simulink model "Test_of_Hover_Controller"  (R2023a)
settings: Solver=FixedStepAuto  StartTime=0.0  StopTime=150  FixedStep=0.001  RelTol=1e-3
libraries: simulink x2
settings Model: Creator=邓宇飞  LastModifiedBy=邓宇飞

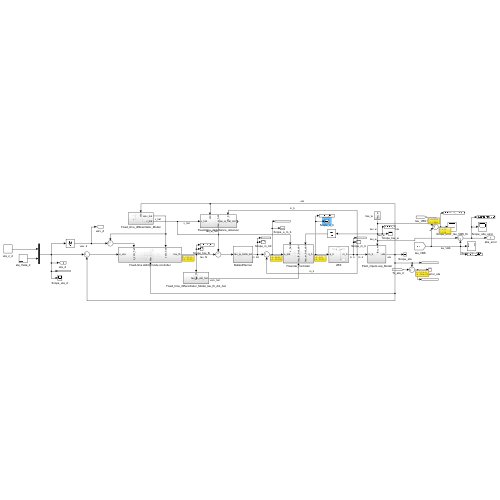
[thumbnail: Simulink's stored preview of the top-level diagram]
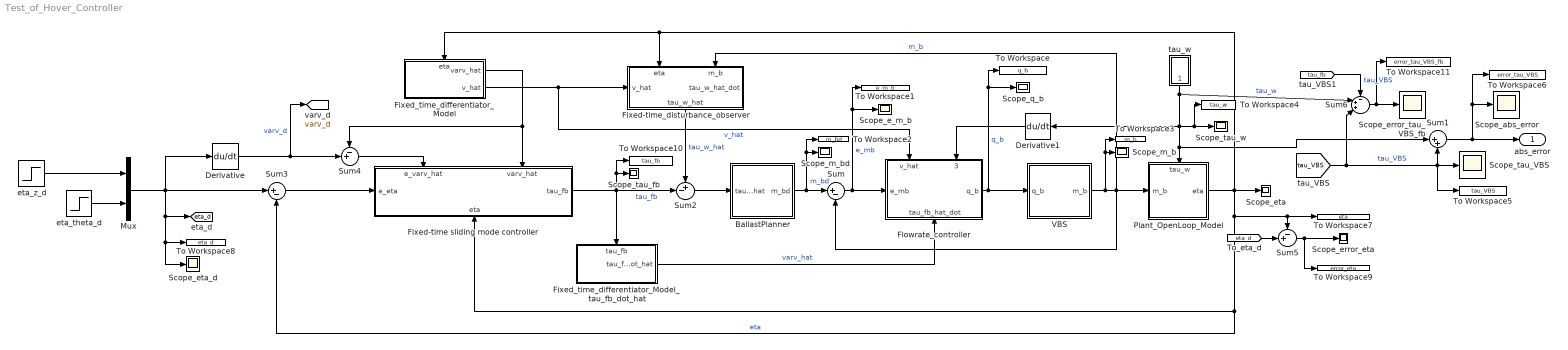
== system Test_of_Hover_Controller ==
  BallastPlanner : Subsystem
  Derivative : Derivative
  Derivative1 : Derivative
  Fixed-time sliding mode controller : Subsystem
      settings: PortSchema="{\"entries\":[{\"content\":{\"sides\":[{\"content\":{\"connectorIds\":[\"In1\"]},\"type\":\"ConnectorPlacement.EquallySpacedRectSide\",\"uuid\":\"f7eec32a-11e5-493e-91a4-aa23e7798835\"},{\"content\":{\"connectorIds\":[\"Out1\"],\"side\":\"RIGHT\"},\"type\":\"ConnectorPlacement.EquallySpacedRectSide\",\"uuid\":\"2b78eec5-73c8-4d02-9319-0fb2d1bcee33\"},{\"content\":{\"connectorIds\":[\"In2\",\"In3\"],\"side\":\"TOP\"},\"type\":\"ConnectorPlacement.EquallySpacedRectSide\",\"uuid\":\"6bb67a89-6549-4a25-872d-286d7aa8440b\"},{\"content\":{\"connectorIds\":[\"In4\"],\"side\":\"BOTTOM\"},\"type\":\"ConnectorPlacement.EquallySpacedRectSide\",\"uuid\":\"a7c480fa-a393-4283-926e-8262b2c36ba1\"}]},\"type\":\"ConnectorPlacement.EquallySpacedConnector\",\"uuid\":\"ac88fafb-ad61-4f2d-a744-8be38b32af3c\"}],\"packageUris\":[\"http://schema.mathworks.com/mf0/Connector/R2020b\"],\"version\":\"1.0\"}"
  Fixed-time_disturbance_observer : Subsystem
      settings: PortSchema="{\"entries\":[{\"content\":{\"sides\":[{\"content\":{\"connectorIds\":[\"In1\"]},\"type\":\"ConnectorPlacement.EquallySpacedRectSide\",\"uuid\":\"977a3149-1921-48fe-b96a-a4ad28c91371\"},{\"content\":{\"connectorIds\":[\"Out1\"],\"side\":\"RIGHT\"},\"type\":\"ConnectorPlacement.EquallySpacedRectSide\",\"uuid\":\"fff94096-65c1-4681-8bdf-eed371b61c52\"},{\"content\":{\"connectorIds\":[\"In2\",\"In3\"],\"side\":\"TOP\"},\"type\":\"ConnectorPlacement.EquallySpacedRectSide\",\"uuid\":\"5bed714d-ab4b-433b-a946-feaea2816cb1\"},{\"content\":{\"connectorIds\":[\"Out2\"],\"side\":\"BOTTOM\"},\"type\":\"ConnectorPlacement.EquallySpacedRectSide\",\"uuid\":\"4ad85521-d335-4ab1-88b6-9b8c0a3b2785\"}]},\"type\":\"ConnectorPlacement.EquallySpacedConnector\",\"uuid\":\"7c33b186-f768-465e-b799-f94ef9fdf411\"}],\"packageUris\":[\"http://schema.mathworks.com/mf0/Connector/R2020b\"],\"version\":\"1.0\"}"
  Fixed_time_differentiator_Model : Subsystem
      settings: PortSchema="{\"entries\":[{\"content\":{\"sides\":[{\"content\":{},\"type\":\"ConnectorPlacement.EquallySpacedRectSide\",\"uuid\":\"99f788c9-d3b5-4afa-bbaa-ac2c57ad12cb\"},{\"content\":{\"connectorIds\":[\"Out1\",\"Out2\"],\"side\":\"RIGHT\"},\"type\":\"ConnectorPlacement.EquallySpacedRectSide\",\"uuid\":\"b4add6d1-b599-4d1a-a211-146e19e09e31\"},{\"content\":{\"connectorIds\":[\"In1\"],\"side\":\"TOP\"},\"type\":\"ConnectorPlacement.EquallySpacedRectSide\",\"uuid\":\"d4aeca70-b9bd-44c3-bfe7-6ab0567a3ae9\"}]},\"type\":\"ConnectorPlacement.EquallySpacedConnector\",\"uuid\":\"acaab675-7958-4b63-89da-846c50cb8508\"}],\"packageUris\":[\"http://schema.mathworks.com/mf0/Connector/R2020b\"],\"version\":\"1.0\"}"
  Fixed_time_differentiator_Model_tau_fb_dot_hat : Subsystem
      settings: PortSchema="{\"entries\":[{\"content\":{\"sides\":[{\"content\":{},\"type\":\"ConnectorPlacement.EquallySpacedRectSide\",\"uuid\":\"509b689f-cae1-4523-9372-2499bd3b7d9d\"},{\"content\":{\"connectorIds\":[\"Out1\"],\"side\":\"RIGHT\"},\"type\":\"ConnectorPlacement.EquallySpacedRectSide\",\"uuid\":\"a1df743b-e6a9-4451-86f2-27990c18dc24\"},{\"content\":{\"connectorIds\":[\"In1\"],\"side\":\"TOP\"},\"type\":\"ConnectorPlacement.EquallySpacedRectSide\",\"uuid\":\"5149f091-ad88-4d80-a39f-36dd9d24fd7a\"},{\"content\":{\"side\":\"BOTTOM\"},\"type\":\"ConnectorPlacement.EquallySpacedRectSide\",\"uuid\":\"b5eefe9f-7883-4d8e-a8af-dce689347657\"}]},\"type\":\"ConnectorPlacement.EquallySpacedConnector\",\"uuid\":\"61175d6f-7ec4-4947-9258-193f13282eb9\"}],\"packageUris\":[\"http://schema.mathworks.com/mf0/Connector/R2020b\"],\"version\":\"1.0\"}"
  Flowrate_controller : Subsystem
      settings: PortSchema="{\"entries\":[{\"content\":{\"sides\":[{\"content\":{\"connectorIds\":[\"In1\"]},\"type\":\"ConnectorPlacement.EquallySpacedRectSide\",\"uuid\":\"977a3149-1921-48fe-b96a-a4ad28c91371\"},{\"content\":{\"connectorIds\":[\"Out1\"],\"side\":\"RIGHT\"},\"type\":\"ConnectorPlacement.EquallySpacedRectSide\",\"uuid\":\"fff94096-65c1-4681-8bdf-eed371b61c52\"},{\"content\":{\"connectorIds\":[\"In2\",\"In3\"],\"side\":\"TOP\"},\"type\":\"ConnectorPlacement.EquallySpacedRectSide\",\"uuid\":\"5bed714d-ab4b-433b-a946-feaea2816cb1\"},{\"content\":{\"connectorIds\":[\"In4\"],\"side\":\"BOTTOM\"},\"type\":\"ConnectorPlacement.EquallySpacedRectSide\",\"uuid\":\"e9124608-fe81-4a90-8a38-d0d96a25662d\"}]},\"type\":\"ConnectorPlacement.EquallySpacedConnector\",\"uuid\":\"7c33b186-f768-465e-b799-f94ef9fdf411\"}],\"packageUris\":[\"http://schema.mathworks.com/mf0/Connector/R2020b\"],\"version\":\"1.0\"}"
  Mux : Mux  Inputs=2
  Plant_OpenLoop_Model : Subsystem
      settings: PortSchema="{\"entries\":[{\"content\":{\"sides\":[{\"content\":{\"connectorIds\":[\"In1\"]},\"type\":\"ConnectorPlacement.EquallySpacedRectSide\",\"uuid\":\"171ab365-2c9c-477f-ab94-6e1b535ce398\"},{\"content\":{\"connectorIds\":[\"Out1\"],\"side\":\"RIGHT\"},\"type\":\"ConnectorPlacement.EquallySpacedRectSide\",\"uuid\":\"68d15153-0085-4baf-9515-c294b6b9b8eb\"},{\"content\":{\"connectorIds\":[\"In2\"],\"side\":\"TOP\"},\"type\":\"ConnectorPlacement.EquallySpacedRectSide\",\"uuid\":\"3f887e7e-8b06-4bf2-b39d-d49324deef58\"},{\"content\":{\"side\":\"BOTTOM\"},\"type\":\"ConnectorPlacement.EquallySpacedRectSide\",\"uuid\":\"0c56d0aa-527a-42c0-aa98-8ee52c9400f1\"}]},\"type\":\"ConnectorPlacement.EquallySpacedConnector\",\"uuid\":\"a8f2799e-4d6b-4adf-9803-c3f607cd4a91\"}],\"packageUris\":[\"http://schema.mathworks.com/mf0/Connector/R2020b\"],\"version\":\"1.0\"}"
  Scope_abs_error : Scope
  Scope_e_m_b : Scope
  Scope_error_eta : Scope
  Scope_error_tau_VBS_fb : Scope
  Scope_eta : Scope
  Scope_eta_d : Scope
  Scope_m_b : Scope
  Scope_m_bd : Scope
  Scope_q_b : Scope
  Scope_tau_VBS : Scope
  Scope_tau_fb : Scope
  Scope_tau_w : Scope
  Sum : Sum  Inputs=|+-
  Sum1 : Sum  Inputs=|++
  Sum2 : Sum  Inputs=+-|
  Sum3 : Sum  Inputs=|+-
  Sum4 : Sum  Inputs=-+|
  Sum5 : Sum  Inputs=-+|
  Sum6 : Sum  Inputs=-++|
  To Workspace : ToWorkspace  VariableName=q_b  SaveFormat=Timeseries  SampleTime=-1
  To Workspace1 : ToWorkspace  VariableName=e_m_b  SaveFormat=Timeseries  SampleTime=-1
  To Workspace10 : ToWorkspace  VariableName=tau_fb  SaveFormat=Timeseries  SampleTime=-1
  To Workspace11 : ToWorkspace  VariableName=error_tau_VBS_fb  SaveFormat=Timeseries  SampleTime=-1
  To Workspace2 : ToWorkspace  VariableName=m_bd  SaveFormat=Timeseries  SampleTime=-1
  To Workspace3 : ToWorkspace  VariableName=m_b  SaveFormat=Timeseries  SampleTime=-1
  To Workspace4 : ToWorkspace  VariableName=tau_w  SaveFormat=Timeseries  SampleTime=-1
  To Workspace5 : ToWorkspace  VariableName=tau_VBS  SaveFormat=Timeseries  SampleTime=-1
  To Workspace6 : ToWorkspace  VariableName=error_tau_VBS  SaveFormat=Timeseries  SampleTime=-1
  To Workspace7 : ToWorkspace  VariableName=eta  SaveFormat=Timeseries  SampleTime=-1
  To Workspace8 : ToWorkspace  VariableName=eta_d  SaveFormat=Timeseries  SampleTime=-1
  To Workspace9 : ToWorkspace  VariableName=error_eta  SaveFormat=Timeseries  SampleTime=-1
  VBS : Subsystem
  eta_theta_d : Step  After=0  SampleTime=0
  eta_z_d : Step  After=0  SampleTime=0
  tau_w : Subsystem
  abs_error : Outport
  tag scope: eta_d=global, varv_d=global
  wires:
  Sum3/1 -> Fixed-time sliding mode controller/1(e_eta)
  eta_theta_d/1 -> Mux/2
  [tau_VBS] -> Sum6/3, Scope_tau_VBS/1, Sum1/2, To Workspace5/1  "tau_VBS"
  eta_z_d/1 -> Mux/1
  Sum/1 -> Flowrate_controller/1(e_mb), To Workspace1/1, Scope_e_m_b/1  "e_mb"
  Fixed_time_differentiator_Model/2(v_hat) -> Flowrate_controller/2(v_hat), Fixed-time_disturbance_observer/1(v_hat)  "v_hat"
  Derivative/1 -> [varv_d], Sum4/2  "varv_d"
  tau_w/1(tau_w) -> Sum6/2, To Workspace4/1, Scope_tau_w/1, Plant_OpenLoop_Model/2(tau_w), Sum1/1, Derivative1/1  "tau_w"
  Sum1/1 -> To Workspace6/1, Scope_abs_error/1, abs_error/1
  VBS/1(m_b) -> To Workspace3/1, Scope_m_b/1, Fixed-time_disturbance_observer/3(m_b), Sum/2, Plant_OpenLoop_Model/1(m_b)  "m_b"
  Flowrate_controller/1(q_b) -> Scope_q_b/1, To Workspace/1, VBS/1(q_b)  "q_b"
  Mux/1 -> Sum3/1, [eta_d], To Workspace8/1, Scope_eta_d/1, Derivative/1
  BallastPlanner/1(m_bd) -> To Workspace2/1, Scope_m_bd/1, Sum/1  "m_bd"
  Fixed-time sliding mode controller/1(tau_fb) -> To Workspace10/1, Scope_tau_fb/1, Fixed_time_differentiator_Model_tau_fb_dot_hat/1(tau_fb), Sum2/2  "tau_fb"
  Fixed-time_disturbance_observer/2(tau_w_hat) -> Sum2/1  "tau_w_hat"
  Sum2/1 -> BallastPlanner/1(tau_w_hat)
  Fixed_time_differentiator_Model_tau_fb_dot_hat/1(tau_fb_dot_hat) -> Flowrate_controller/4(tau_fb_hat_dot)  "varv_hat"
  Plant_OpenLoop_Model/1(eta) -> To Workspace7/1, Sum5/1, Fixed-time sliding mode controller/4(eta), Sum3/2, Scope_eta/1, Fixed_time_differentiator_Model/1(eta), Fixed-time_disturbance_observer/2(eta)  "eta"
  Fixed_time_differentiator_Model/1(varv_hat) -> Fixed-time sliding mode controller/3(varv_hat), Sum4/1
  Sum4/1 -> Fixed-time sliding mode controller/2(e_varv_hat)
  Derivative1/1 -> Flowrate_controller/3(tau_w_hat_dot)
  [eta_d] -> Sum5/2
  Sum5/1 -> To Workspace9/1, Scope_error_eta/1
  [tau_fb] -> Sum6/1  "tau_VBS"
  Sum6/1 -> To Workspace11/1, Scope_error_tau_VBS_fb/1

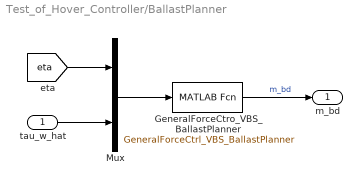
== system Test_of_Hover_Controller/BallastPlanner ==
  tau_w_hat : Inport
  GeneralForceCtro_VBS_BallastPlanner : MATLABFcn  MATLABFcn=GeneralForceCtrl_VBS_BallastPlanner  OutputDimensions=2  OutputSignalType=real
  Mux : Mux  Inputs=2
  m_bd : Outport
  wires:
  Mux/1 -> GeneralForceCtro_VBS_BallastPlanner/1
  GeneralForceCtro_VBS_BallastPlanner/1 -> m_bd/1  "m_bd"
  [eta] -> Mux/1
  tau_w_hat/1 -> Mux/2

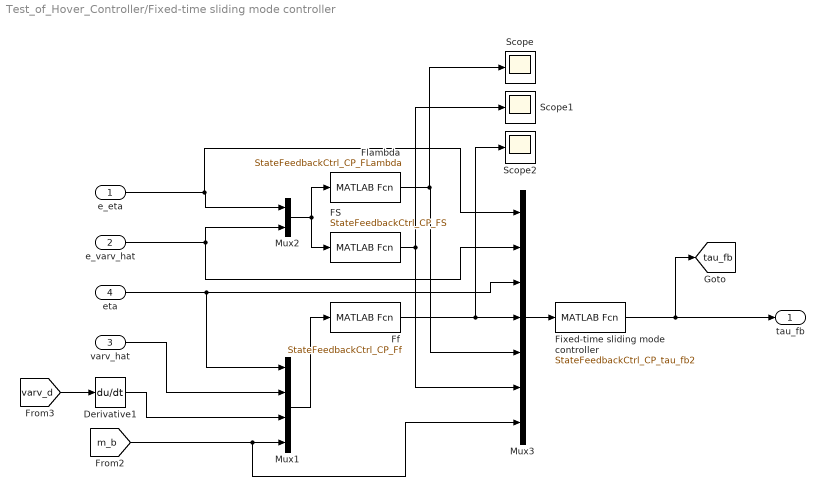
== system Test_of_Hover_Controller/Fixed-time sliding mode controller ==
  e_eta : Inport
  e_varv_hat : Inport  Port=2
  varv_hat : Inport  Port=3
  eta : Inport  Port=4
  Derivative1 : Derivative
  FS : MATLABFcn  MATLABFcn=StateFeedbackCtrl_CP_FS  OutputDimensions=2  OutputSignalType=real
  Ff : MATLABFcn  MATLABFcn=StateFeedbackCtrl_CP_Ff  OutputDimensions=2  OutputSignalType=real
  Fixed-time sliding mode controller : MATLABFcn  MATLABFcn=StateFeedbackCtrl_CP_tau_fb2  OutputDimensions=2  OutputSignalType=real
  Flambda : MATLABFcn  MATLABFcn=StateFeedbackCtrl_CP_FLambda  OutputDimensions=2  OutputSignalType=real
  Mux1 : Mux
  Mux2 : Mux  Inputs=2
  Mux3 : Mux  Inputs=7
  Scope : Scope
  Scope1 : Scope
  Scope2 : Scope
  tau_fb : Outport
  tag scope: tau_fb=global
  wires:
  eta/1 -> Mux3/3, Mux1/1
  e_varv_hat/1 -> Mux2/2, Mux3/2
  e_eta/1 -> Mux3/1, Mux2/1
  Mux2/1 -> Flambda/1, FS/1
  FS/1 -> Scope1/1, Mux3/6
  Flambda/1 -> Scope/1, Mux3/5
  Ff/1 -> Scope2/1, Mux3/4
  Mux1/1 -> Ff/1
  [m_b] -> Mux3/7, Mux1/4
  Mux3/1 -> Fixed-time sliding mode controller/1
  varv_hat/1 -> Mux1/2
  Derivative1/1 -> Mux1/3
  [varv_d] -> Derivative1/1
  Fixed-time sliding mode controller/1 -> tau_fb/1, [tau_fb]

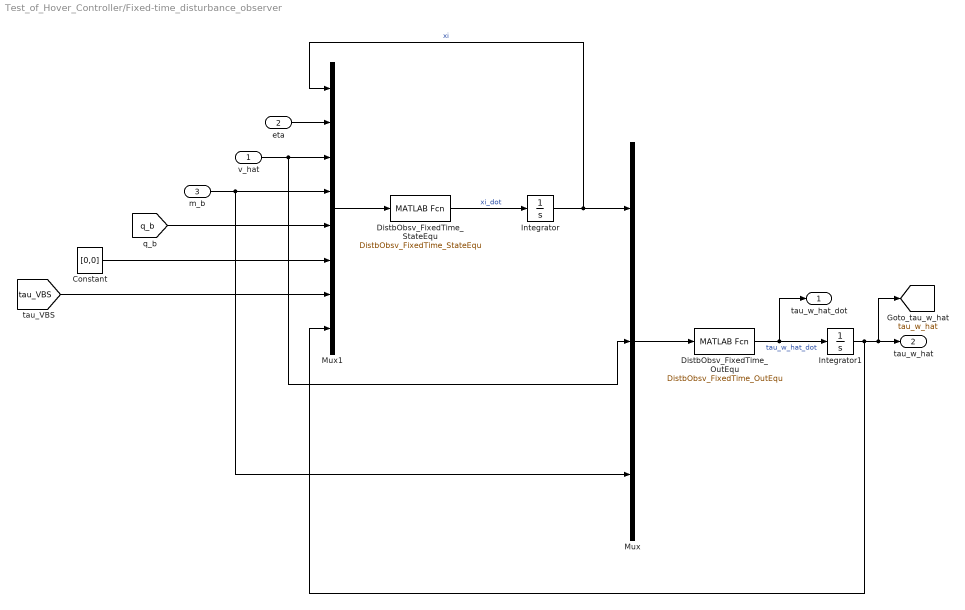
== system Test_of_Hover_Controller/Fixed-time_disturbance_observer ==
  v_hat : Inport
  eta : Inport  Port=2
  m_b : Inport  Port=3
  Constant : Constant  Value=[0,0]
  DistbObsv_FixedTime_OutEqu : MATLABFcn  MATLABFcn=DistbObsv_FixedTime_OutEqu  OutputDimensions=2  OutputSignalType=real
  DistbObsv_FixedTime_StateEqu : MATLABFcn  MATLABFcn=DistbObsv_FixedTime_StateEqu  OutputDimensions=2  OutputSignalType=real
  Integrator : Integrator
  Integrator1 : Integrator
  Mux : Mux  Inputs=3
  Mux1 : Mux  Inputs=8
  tau_w_hat_dot : Outport
  tau_w_hat : Outport  Port=2
  tag scope: tau_w_hat=global
  wires:
  Integrator1/1 -> [tau_w_hat], tau_w_hat/1, Mux1/8
  Integrator/1 -> Mux1/1, Mux/1  "xi"
  DistbObsv_FixedTime_OutEqu/1 -> tau_w_hat_dot/1, Integrator1/1  "tau_w_hat_dot"
  Mux/1 -> DistbObsv_FixedTime_OutEqu/1
  Mux1/1 -> DistbObsv_FixedTime_StateEqu/1
  DistbObsv_FixedTime_StateEqu/1 -> Integrator/1  "xi_dot"
  eta/1 -> Mux1/2
  v_hat/1 -> Mux/2, Mux1/3
  m_b/1 -> Mux/3, Mux1/4
  [q_b] -> Mux1/5
  Constant/1 -> Mux1/6
  [tau_VBS] -> Mux1/7

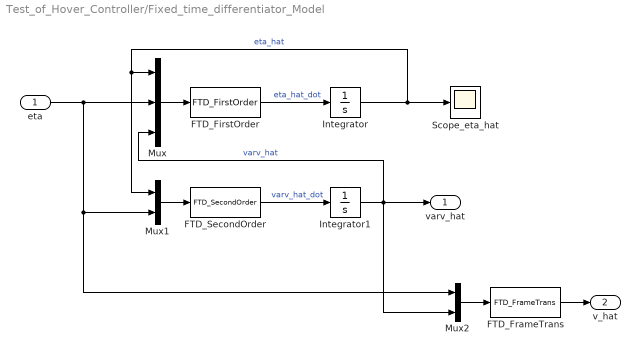
== system Test_of_Hover_Controller/Fixed_time_differentiator_Model ==
  eta : Inport
  FTD_FirstOrder : MATLABFcn  MATLABFcn=FTD_FirstOrder  OutputDimensions=2  OutputSignalType=real
  FTD_FrameTrans : MATLABFcn  MATLABFcn=FTD_FrameTrans  OutputDimensions=2  OutputSignalType=real
  FTD_SecondOrder : MATLABFcn  MATLABFcn=FTD_SecondOrder  OutputDimensions=2  OutputSignalType=real
  Integrator : Integrator
  Integrator1 : Integrator
  Mux : Mux  Inputs=3
  Mux1 : Mux  Inputs=2
  Mux2 : Mux  Inputs=2
  Scope_eta_hat : Scope
  varv_hat : Outport
  v_hat : Outport  Port=2
  wires:
  Integrator1/1 -> Mux2/2, varv_hat/1, Mux/3  "varv_hat"
  eta/1 -> Mux2/1, Mux1/2, Mux/2
  FTD_SecondOrder/1 -> Integrator1/1  "varv_hat_dot"
  FTD_FrameTrans/1 -> v_hat/1
  FTD_FirstOrder/1 -> Integrator/1  "eta_hat_dot"
  Integrator/1 -> Mux1/1, Mux/1, Scope_eta_hat/1  "eta_hat"
  Mux/1 -> FTD_FirstOrder/1
  Mux2/1 -> FTD_FrameTrans/1
  Mux1/1 -> FTD_SecondOrder/1

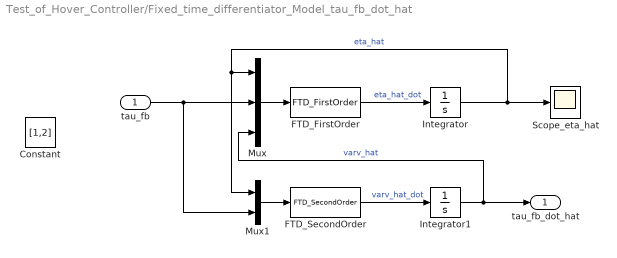
== system Test_of_Hover_Controller/Fixed_time_differentiator_Model_tau_fb_dot_hat ==
  tau_fb : Inport
  Constant : Constant  Value=[1,2]
  FTD_FirstOrder : MATLABFcn  MATLABFcn=FTD_FirstOrder  OutputDimensions=2
  FTD_SecondOrder : MATLABFcn  MATLABFcn=FTD_SecondOrder  OutputDimensions=2
  Integrator : Integrator
  Integrator1 : Integrator
  Mux : Mux  Inputs=3
  Mux1 : Mux  Inputs=2
  Scope_eta_hat : Scope
  tau_fb_dot_hat : Outport
  wires:
  Integrator/1 -> Mux1/1, Mux/1, Scope_eta_hat/1  "eta_hat"
  Integrator1/1 -> tau_fb_dot_hat/1, Mux/3  "varv_hat"
  Mux/1 -> FTD_FirstOrder/1
  Mux1/1 -> FTD_SecondOrder/1
  FTD_SecondOrder/1 -> Integrator1/1  "varv_hat_dot"
  FTD_FirstOrder/1 -> Integrator/1  "eta_hat_dot"
  tau_fb/1 -> Mux1/2, Mux/2

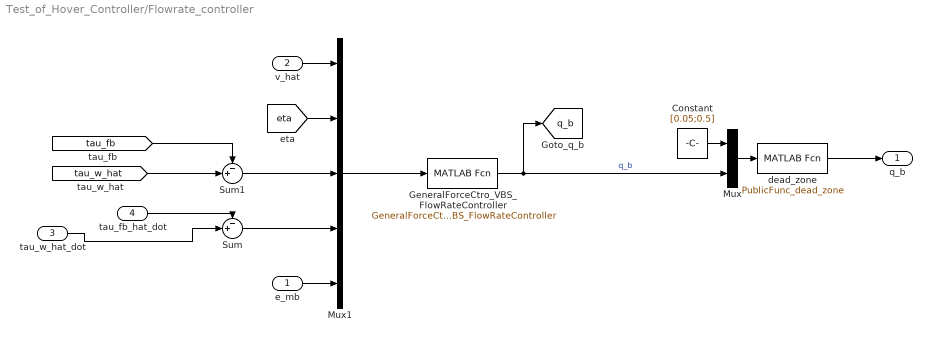
== system Test_of_Hover_Controller/Flowrate_controller ==
  e_mb : Inport
  v_hat : Inport  Port=2
  tau_w_hat_dot : Inport  Port=3
  tau_fb_hat_dot : Inport  Port=4
  Constant : Constant  Value=[0.05;0.5]
  GeneralForceCtro_VBS_FlowRateController : MATLABFcn  MATLABFcn=GeneralForceCtrl_VBS_FlowRateController  OutputDimensions=2  OutputSignalType=real
  Mux : Mux  Inputs=2
  Mux1 : Mux  Inputs=5
  Sum : Sum  Inputs=-+|
  Sum1 : Sum  Inputs=-+|
  dead_zone : MATLABFcn  MATLABFcn=PublicFunc_dead_zone  OutputDimensions=2  OutputSignalType=real
  q_b : Outport
  tag scope: q_b=global
  wires:
  Mux1/1 -> GeneralForceCtro_VBS_FlowRateController/1
  GeneralForceCtro_VBS_FlowRateController/1 -> [q_b], Mux/2  "q_b"
  v_hat/1 -> Mux1/1
  [eta] -> Mux1/2
  Sum/1 -> Mux1/4
  e_mb/1 -> Mux1/5
  tau_w_hat_dot/1 -> Sum/2
  tau_fb_hat_dot/1 -> Sum/1
  dead_zone/1 -> q_b/1
  Mux/1 -> dead_zone/1
  Constant/1 -> Mux/1
  [tau_w_hat] -> Sum1/2
  Sum1/1 -> Mux1/3
  [tau_fb] -> Sum1/1

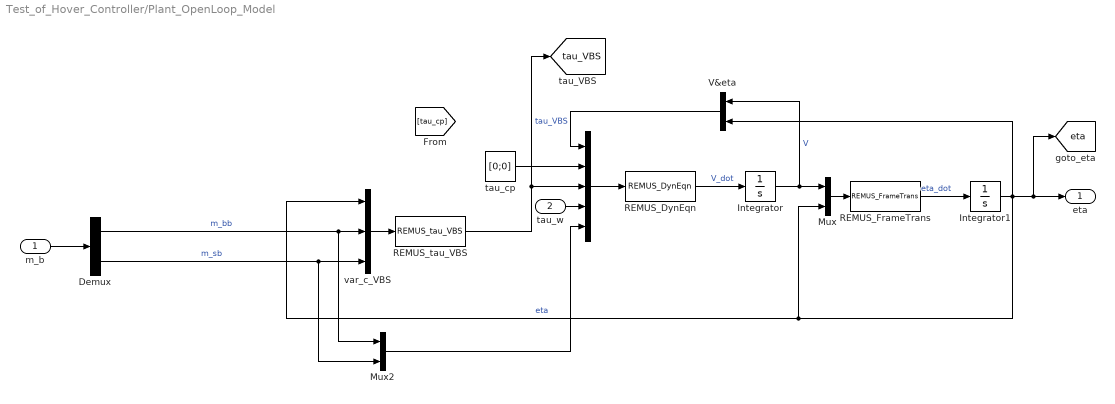
== system Test_of_Hover_Controller/Plant_OpenLoop_Model ==
  m_b : Inport
  tau_w : Inport  Port=2
  " " : Mux  Inputs=5
  Demux : Demux  Outputs=2
  Integrator : Integrator
  Integrator1 : Integrator
  Mux : Mux  Inputs=2
  Mux2 : Mux  Inputs=2
  REMUS_DynEqn : MATLABFcn  MATLABFcn=REMUS_DynEqn  OutputDimensions=2
  REMUS_FrameTrans : MATLABFcn  MATLABFcn=REMUS_FrameTrans  OutputDimensions=2
  REMUS_tau_VBS : MATLABFcn  MATLABFcn=REMUS_tau_VBS  OutputDimensions=2
  V&eta : Mux  Inputs=2
  tau_cp : Constant  Value=[0;0]
  var_c_VBS : Mux  Inputs=3
  eta : Outport
  tag scope: eta=global, tau_VBS=global
  wires:
  REMUS_DynEqn/1 -> Integrator/1  "V_dot"
  Integrator1/1 -> [eta], eta/1, Mux/2, var_c_VBS/1, V&eta/2  "eta"
  Demux/2 -> Mux2/2, var_c_VBS/3  "m_sb"
  Mux/1 -> REMUS_FrameTrans/1
  " "/1 -> REMUS_DynEqn/1
  Integrator/1 -> Mux/1, V&eta/1  "V"
  Demux/1 -> Mux2/1, var_c_VBS/2  "m_bb"
  V&eta/1 -> " "/1
  REMUS_tau_VBS/1 -> [tau_VBS], " "/3  "tau_VBS"
  tau_w/1 -> " "/4
  REMUS_FrameTrans/1 -> Integrator1/1  "eta_dot"
  var_c_VBS/1 -> REMUS_tau_VBS/1
  Mux2/1 -> " "/5
  m_b/1 -> Demux/1
  tau_cp/1 -> " "/2

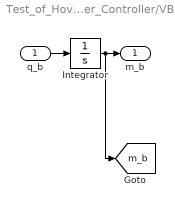
== system Test_of_Hover_Controller/VBS ==
  q_b : Inport
  Integrator : Integrator
  m_b : Outport
  tag scope: m_b=global
  wires:
  q_b/1 -> Integrator/1
  Integrator/1 -> [m_b], m_b/1

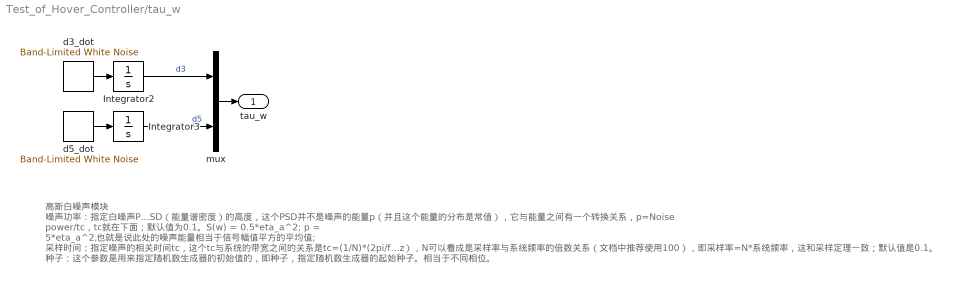
== system Test_of_Hover_Controller/tau_w ==
  note: 高斯白噪声模块
      | 噪声功率：指定白噪声PSD（能量谱密度）的高度，这个PSD并不是噪声的能量p（并且这个能量的分布是常值），它与能量之间有一个转换关系，p=Noise power/tc，tc就在下面；默认值为0.1。S(w) = 0.5*eta_a^2;
      | p = 5*eta_a^2;也就是说此处的噪声能量相当于信号幅值平方的平均值;
      | 采样时间：指定噪声的相关时间tc，这个tc与系统的带宽之间的关系是tc=(1/N)*(2pi/fmax)，其中fmax是系统的带宽（实际上是角频率，fmax=2*pi*f，这个f才是我们常使用的频率Hz），N可以看成是采样率与系统频率的倍数关系（文档中推荐使用100），即采样率=N*系统频率，这和采样定理一致；默认值是0.1。
      | 种子：这个参数是用来指定随机数生成器的初始值的，即种子，指定随机数生成器的起始种子。相当于不同相位。
  Integrator2 : Integrator
  Integrator3 : Integrator
  d3_dot : simulink/Sources/Band-Limited White Noise  Cov=[0.5]  Ts=0.1  seed=[2]
  d5_dot : simulink/Sources/Band-Limited White Noise  Cov=[0.1]  Ts=0.1  seed=[3]
  mux : Mux  Inputs=2
  tau_w : Outport
  wires:
  Integrator3/1 -> mux/2  "d5"
  d5_dot/1 -> Integrator3/1
  d3_dot/1 -> Integrator2/1
  mux/1 -> tau_w/1
  Integrator2/1 -> mux/1  "d3"
